simulink model "sf_cpp"  (Simulink 7.6)
settings: Solver=FixedStepDiscrete  StartTime=0.0  StopTime=inf  RelTol=1e-3
settings Model: Creator=The MathWorks Inc.  CovMetricSettings=dcmtr  ExtModeAutoUpdateStatusClock=off
settings DataIOCC: SaveOutput=off  SaveTime=off  SignalLoggingName=sigsOut
settings OptimizationCC: InlineParams=on  InlineInvariantSignals=on  StateBitsets=on  DataBitsets=on  UseTempVars=on  InitFltsAndDblsToZero=on  BufferReusableBoundary=off
settings DebuggingCC: SaveWithParameterizedLinksMsg=none  CheckExecutionContextPreStartOutputMsg=on  CheckExecutionContextRuntimeOutputMsg=on  SignalResolutionControl=TryResolveAllWithWarning  SolverPrmCheckMsg=none  MultiTaskDSMMsg=warning  MultiTaskCondExecSysMsg=none  StrictBusMsg=None
settings HardwareCC: TargetHWDeviceType=32-bit Generic
settings SFSimCC: SimCustomHeaderCode="#include \"adder_cpp.h\""  SimCustomInitializer=adderVar = createAdder();  SimCustomTerminator=deleteAdder(adderVar);  SimUserSources=./custom_cpp_src/adder_cpp.cpp  SimUserIncludeDirs=./custom_cpp_src  SimParseCustomCode=off
settings RTWCC: GenerateReport=on  RTWVerbose=off  CustomSourceCode="#include \"adder_cpp.h\""  CustomInclude=./custom_cpp_src  CustomSource=./custom_cpp_src/adder_cpp.cpp  CustomInitializer=adderVar = createAdder();  CustomTerminator=deleteAdder(adderVar);  LaunchReport=on  TargetLang=C++  IncludeERTFirstTime=on
settings CodeAppCC: ForceParamTrailComments=on
settings GRTTargetCC: TargetFcnLib=ansi_tfl_tmw.mat

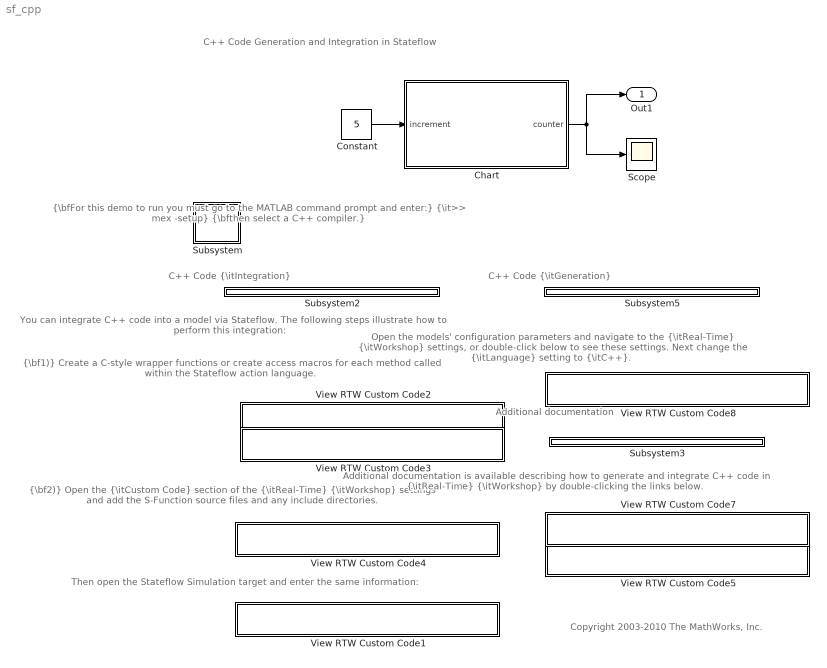
== system sf_cpp ==
  note: Then open the Stateflow Simulation target
      | and enter the same information:
  note: {\bf1)} Create a C-style wrapper functions or
      |      create access macros for each method
      |      called within the Stateflow action language.
  note: {\bfFor this demo to run you must go to the MATLAB command prompt and enter:} {\it>> mex -setup}
      | {\bfthen select a C++ compiler.}
  note: C++ Code {\itIntegration}
  note: You can integrate C++ code into a model via
      | Stateflow.  The following steps illustrate
      | how to perform this integration:
  note: {\bf2)} Open the {\itCustom Code} section
      |      of the {\itReal-Time} {\itWorkshop} settings and
      |      add the S-Function source files and any
      |      include directories.
  note: C++ Code Generation and Integration in Stateflow
  note: Additional documentation
  note: Additional documentation is available
      | describing how to generate and integrate
      | C++ code in {\itReal-Time} {\itWorkshop}
      | by double-clicking the links below.
  note: Open the models' configuration parameters
      | and navigate to the {\itReal-Time} {\itWorkshop}
      | settings, or double-click below to see these
      | settings.  Next change the {\itLanguage} setting
      | to {\itC++}.
  note: C++ Code {\itGeneration}
  note: Copyright 2003-2010 The MathWorks, Inc.
  Chart : Stateflow chart  TreatAsAtomicUnit=on
  Constant : Constant  Value=5
  Scope : Scope
      settings: YMin=15  YMax=105
  Subsystem : Subsystem
      mask init:
      | pos    = get_param(gcb, 'Position');
      | width  = pos(3) - pos(1);
      | height = pos(4) - pos(2);
      | 
      | marginPercent = 20;
      | marginPixels  = round(marginPercent / 100 * width);
      | 
      | x1 = width - marginPixels;
      | y1 = height;
      | x2 = width;
      | y2 = height - marginPixels;
      | x3 = width;
      | y3 = marginPixels;
      | x4 = width - marginPixels;
      | y4 = 0;
      | x5 = marginPixels;
      | y5 = 0;
      | x6 = 0;
      | y6 = marginPixels;
      | x7 = 0;
      | y7 = height - marginPixels;
      | x8 = marginPixels;
      | y8 = height;
      | 
      | xvec = [x1, x2, x3, x4, x5, x6, x7, x8];
      | yvec = [y1, y2, y3, y4, y5, y6, y7, y8];
      mask Display:
      | color('red');
      | patch(xvec, yvec);
      | color('white');
      | disp('!');
  Subsystem2 : Subsystem
  Subsystem3 : Subsystem
  Subsystem5 : Subsystem
  View RTW Custom Code1 : Subsystem
      mask init:
      | pos    = get_param(gcb, 'Position');
      | width  = pos(3) - pos(1);
      | height = pos(4) - pos(2);
      | 
      | 
      | % Compute arrow coordinates
      | arrowW = width  / 20;
      | arrowH = height / 2.5;
      | arrowX = width  / 50;
      | arrowY = height / 3;
      | arrowXvec = [arrowX, arrowX, arrowX + arrowW];
      | arrowYvec = [arrowY, arrowY + arrowH, arrowY + arrowH / 2];
      | 
      | % Compute text position
      | textXbuff = width / 30;
      | textX  = arrowX + arrowW + textXbuff;
      | textY  = height / 2;
      settings: NameChangeFcn=|
      | model = bdroot;
      | slCfgPrmDlg(model,'Open');
      | slCfgPrmDlg(bdroot,'TurnToPage','Simulation Target/Custom Code');
      | clear model;
      settings: OpenFcn=|
      | model = bdroot;
      | slCfgPrmDlg(model,'Open');
      | slCfgPrmDlg(bdroot,'TurnToPage','Simulation Target/Custom Code');
      | clear model;
      mask Display:
      | patch(arrowXvec, arrowYvec);
      | text(textX, textY, 'Open Stateflow Simulation Target');
  View RTW Custom Code2 : Subsystem
      mask init: same as sf_cpp/View RTW Custom Code1
      settings: OpenFcn=|
      | filename=fullfile(matlabroot, 'toolbox', 'stateflow', 'sfdemos', 'custom_cpp_src', 'adder_cpp.cpp');
      | eval('edit(filename)')
      mask Display:
      | patch(arrowXvec, arrowYvec);
      | text(textX, textY, 'Open adder_cpp.cpp');
  View RTW Custom Code3 : Subsystem
      mask init: same as sf_cpp/View RTW Custom Code1
      settings: OpenFcn=|
      | filename=fullfile(matlabroot, 'toolbox', 'stateflow', 'sfdemos', 'custom_cpp_src', 'adder_cpp.h');
      | eval('edit(filename)')
      mask Display:
      | patch(arrowXvec, arrowYvec);
      | text(textX, textY, 'Open adder_cpp.h');
  View RTW Custom Code4 : Subsystem
      mask init: same as sf_cpp/View RTW Custom Code1
      settings: OpenFcn=|
      | model = bdroot;
      | slCfgPrmDlg(model,'Open');
      | slCfgPrmDlg(bdroot,'TurnToPage','Real-Time Workshop/Custom Code');
      | clear model;
      mask Display:
      | patch(arrowXvec, arrowYvec);
      | text(textX, textY, 'Open Custom Code Settings');
  View RTW Custom Code5 : Subsystem
      mask init: same as sf_cpp/View RTW Custom Code1
      settings: OpenFcn=helpview([docroot '/toolbox/rtw/helptargets.map'], 'rtw_cpp_limitations')
      mask Display:
      | patch(arrowXvec, arrowYvec);
      | text(textX, textY, 'C++ Limitations');
  View RTW Custom Code7 : Subsystem
      mask init: same as sf_cpp/View RTW Custom Code1
      settings: OpenFcn=helpview([docroot '/toolbox/rtw/helptargets.map'], 'rtw_language_support')
      mask Display:
      | patch(arrowXvec, arrowYvec);
      | text(textX, textY, 'C++ Documentation');
  View RTW Custom Code8 : Subsystem
      mask init: same as sf_cpp/View RTW Custom Code1
      settings: OpenFcn=|
      | model = bdroot;
      | slCfgPrmDlg(model,'Open');
      | slCfgPrmDlg(bdroot,'TurnToPage','Real-Time Workshop');
      | clear model;
      mask Display:
      | patch(arrowXvec, arrowYvec);
      | text(textX, textY, 'Open Real-Time Workshop Settings');
  Out1 : Outport
  wires:
  Constant/1 -> Chart/1(increment)
  Chart/1(counter) -> Scope/1, Out1/1

== system sf_cpp/Subsystem ==

== system sf_cpp/Subsystem2 ==

== system sf_cpp/Subsystem3 ==

== system sf_cpp/Subsystem5 ==

== system sf_cpp/View RTW Custom Code1 ==

== system sf_cpp/View RTW Custom Code2 ==

== system sf_cpp/View RTW Custom Code3 ==

== system sf_cpp/View RTW Custom Code4 ==

== system sf_cpp/View RTW Custom Code5 ==

== system sf_cpp/View RTW Custom Code7 ==

== system sf_cpp/View RTW Custom Code8 ==

== stateflow chart Chart ==
  state under_100
    during: counter = adderOutput(adderVar, increment);
  state over_100
    during: counter = adderOutput(adderVar, -increment);
  (default) -> under_100 : / counter = 0;
  under_100 -> over_100 : [counter > 100]
  over_100 -> under_100 : [counter < 0]
  data: increment input int32; counter output double
